simulink model "BEVplantModel"  (R2022b)
settings: Solver=daessc  StartTime=0  StopTime=50  RelTol=1e-3
PreLoadFcn:
  | % Load all parameters
  | BEVplantModelParam;
undefined symbols (not defined in the file): battery, cabin_T_init, coolant_pipe_D, coolant_valve_D_ratio_max, coolant_valve_D_ratio_min, coolant_valve_displacement, electricDrive, max_torque, vehicle, vehicleThermal
libraries: fl_lib x292, nesl_utility x67, SimscapeFluids_lib x15, ee_lib x11, sdl_lib x8, BatteryCurrentManagement x3, slpidlib x3, simulink x2, BatteryThermalManagement x1, autolibshared x1
(part 1 of 10)
Description:
  | Copyright 2022 - 2023 The MathWorks, Inc.
settings Model: PauseTimes=0.4  Creator=jjha  LastModifiedBy=jjha
settings SolverCC: ZeroCrossAlgorithm=Adaptive  DecoupledContinuousIntegration=on
settings DataIOCC: Decimation=10  ReturnWorkspaceOutputs=off  ReturnWorkspaceOutputsName=SimlogBEVdata
settings DebuggingCC: IgnoredZcDiagnostic=none
settings SimscapeCC: SimscapeLogType=all  SimscapeLogSimulationStatistics=on  SimscapeLogToSDI=on  SimscapeLogName=simlogBevPlantModel  SimscapeLogDecimation=10  SimscapeLogLimitData=off

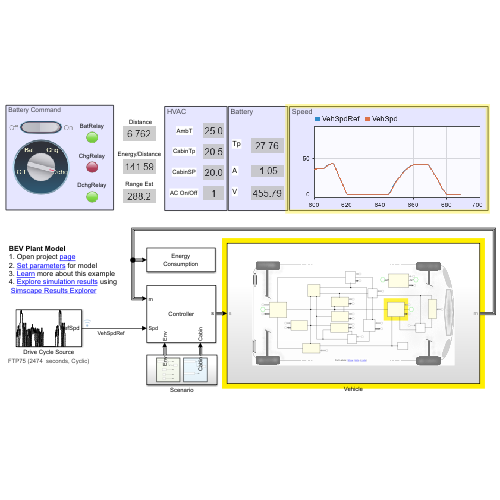
[thumbnail: Simulink's stored preview of the top-level diagram]
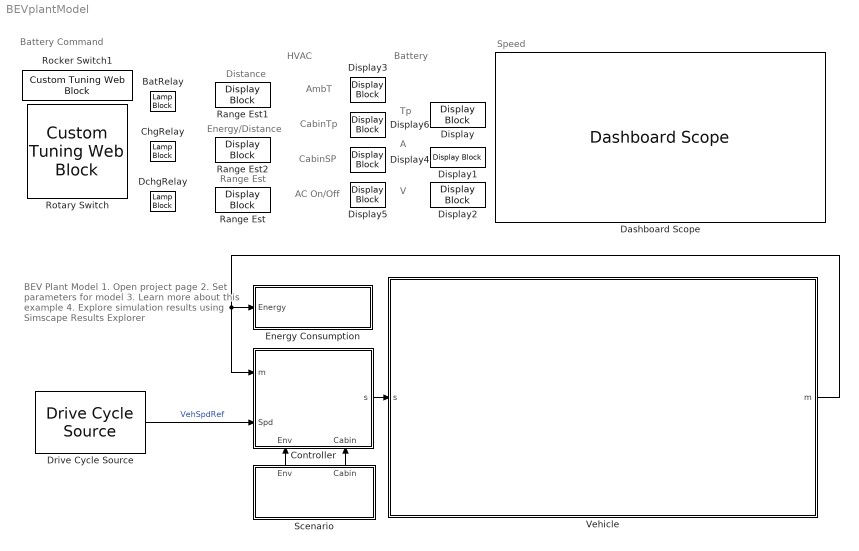
== system BEVplantModel ==
  note: BEV Plant Model
      | 1. Open project page
      | 2. Set parameters for model
      | 3. Learn more about this example
      | 4. Explore simulation results using
      | Simscape Results Explorer
  note: AC On/Off
  note: CabinSP
  note: AmbT
  note: Range Est
  note: HVAC
  note: Tp
  note: Battery
  note: Speed
  note: A
  note: V
  note: CabinTp
  note: Distance
  note: Energy/Distance
  note: Battery Command
  BatRelay : LampBlock  LabelPosition=Hide
  ChgRelay : LampBlock  LabelPosition=Hide
  Controller : Subsystem
      settings: PortSchema="{\"entries\":[{\"content\":{\"sides\":[{\"content\":{\"connectorIds\":[\"In1\",\"In2\"]},\"type\":\"ConnectorPlacement.EquallySpacedRectSide\",\"uuid\":\"c1a23be5-b2bd-489c-89d3-d8ff166adbae\"},{\"content\":{\"connectorIds\":[\"Out1\"],\"side\":\"RIGHT\"},\"type\":\"ConnectorPlacement.EquallySpacedRectSide\",\"uuid\":\"158e6e89-d1bb-4c90-8b36-55bfa29ba4ac\"},{\"content\":{\"connectorIds\":[],\"side\":\"TOP\"},\"type\":\"ConnectorPlacement.EquallySpacedRectSide\",\"uuid\":\"911e2005-fcf6-44eb-a0ec-ba245b30b3ee\"},{\"content\":{\"connectorIds\":[\"In3\",\"In4\"],\"side\":\"BOTTOM\"},\"type\":\"ConnectorPlacement.EquallySpacedRectSide\",\"uuid\":\"99a46f53-b2c3-4e95-9f3e-50b925639021\"}]},\"type\":\"ConnectorPlacement.EquallySpacedConnector\",\"uuid\":\"b6f9d50f-1ffb-42a1-8725-4930e4702b55\"}],\"packageUris\":[\"http://schema.mathworks.com/mf0/Connector/R2020b\"],\"version\":\"1.0\"}"
      mask Display: disp(get_param(gcb, 'Name'))
  Dashboard Scope : DashboardScope  Ymin=0  Ymax=150
  DchgRelay : LampBlock  LabelPosition=Hide
  Display : DisplayBlock  LabelPosition=Hide  Format=Custom  Transparency=1  FormatString=%.2f
  Display1 : DisplayBlock  LabelPosition=Hide  Format=Custom  Transparency=1  FormatString=%.2f
  Display2 : DisplayBlock  LabelPosition=Hide  Format=Custom  Transparency=1  FormatString=%.2f
  Display3 : DisplayBlock  LabelPosition=Hide  Format=Custom  Transparency=1  FormatString=%.1f
  Display4 : DisplayBlock  LabelPosition=Hide  Format=Custom  Transparency=1  FormatString=%.1f
  Display5 : DisplayBlock  LabelPosition=Hide  Format=Integer  Transparency=1  FormatString=%.2f
  Display6 : DisplayBlock  LabelPosition=Hide  Format=Custom  Transparency=1  FormatString=%.1f
  Drive Cycle Source : autolibshared/Drive Cycle Source  cycleVar=FTP75  wsVar=DriveCycleEPA  fileVar=cycleFTP75.mat  tfinal="2474  seconds, Cyclic"  cycleRepeat=on  outAccPort=off  outGearPort=off  gearList=No gear data  t_wot1=5  xdot_woto=0  xdot_wot1=30  t_wot2=20  xdot_wot2=0  t_wotend=30  srcUnit=m/s  outUnit=km/h  srcAccUnit=m/s/s  outAccUnit=m/s^2  dt=0  aMode=1  faultOption=off  velBnd=2  velBndUnit=mph  inUnit=m/s  timeBnd=1  failOption=off  stopSim=off  maxFaultCnt=10  maxFaultTime=2  maxTotFaultTime=15  traceOption=off  dtTrace=1  traceWindow=10  lastDCname=FTP75  lastOutUnit=mph  lastDT=0  lastTB=1  lastSB=2  forceCalcBound=off
  Energy Consumption : Subsystem
      mask Display: disp(get_param(gcb, 'Name'))
  Range Est : DisplayBlock  LabelPosition=Hide  Format=Custom  Transparency=1  FormatString=%.1f
  Range Est1 : DisplayBlock  LabelPosition=Hide  Format=Custom  Transparency=1  FormatString=%.3f
  Range Est2 : DisplayBlock  LabelPosition=Hide  Format=Custom  Transparency=1  FormatString=%.2f
  Rocker Switch1 : CustomTuningWebBlock  LabelPosition=Hide  ShowInitialText=on  Configuration="{\"components\":[{\"name\":\"CustomSwitchStateComponent\",\"settings\":{\"position\":[0,0,1,1],\"states\":[{\"HitRegion\":{\"position\":[0,0,0.5,1]},\"Image\":{\"position\":[0.13,0,1,0.75],\"size\":[1,0.75],\"src\":\"data:image\\/svg+xml;base64,PHN2ZyB4bWxucz0iaHR0cDovL3d3dy53My5vcmcvMjAwMC9zdmciIHhtbG5zOnhsaW5rPSJodHRwOi8vd3d3LnczLm9yZy8xOTk5L3hsaW5rIiB2aWV3Qm94PSIwIDAgNzUgMjQuOCI+PGRlZnM+PHN0eWxlPi5jbHMtMXtmaWxsOnVybCgjcmFkaWFsLWdyYWRpZW50KTt9LmNscy0ye2ZpbGw6dXJsKCNyYWRpYWwtZ3JhZGllbnQtMik7fS5jbHMtM3tzdHJva2U6I2IyMDAwMDtzdHJva2Utd2lkdGg6MC4yNXB4O2ZpbGw6dXJsKCNsaW5lYXItZ3JhZGllbnQpO30uY2xzLTR7ZmlsbDp1cmwoI2xpbmVhci1ncmFkaWVudC0yKTt9LmNs ...(+3576 chars)\",\"srcOrientation\":\"Right\"},\"Label\":{\"color\":[0.5019607843137255,0.5019607843137255,0.5019607843137255],\"icon\":{\"size\":[0,0],\"src\":[],\"srcOrientation\":\"Right\"},\"iconPlacement\":\"left\",\"opacity\":1,\"position\":[0.5,0.08],\"show\":true,\"text\":{\"content\":\"Off\",\"font\":\"Helvetica\",\"fontSize\":14}},\"Value\":0},{\"HitRegion\":{\"position\":[0,0.5,0.5,1]},\"Image\":{\"position\":[0.13,0,1,0.75],\"size\":[1,0.75],\"src\":\"data:image\\/svg+xml;base64,PHN2ZyB4bWxucz0iaHR0cDovL3d3dy53My5vcmcvMjAwMC9zdmciIHhtbG5zOnhsaW5rPSJodHRwOi8vd3d3LnczLm9yZy8xOTk5L3hsaW5rIiB2aWV3Qm94PSIwIDAgNzUgMjQuOCI+PGRlZnM+PHN0eWxlPi5jbHMtMXtmaWxsOnVybCgjcmFkaWFsLWdyYWRpZW50KTt9LmNscy0ye2ZpbGw6dXJsKCNyYWRpYWwtZ3JhZGllbnQtMik7fS5jbHMtM3tzdHJva2U6I2IyMDAwMDtzdHJva2Utd2lkdGg6MC4yNXB4O2ZpbGw6dXJsKCNsaW5lYXItZ3JhZGllbnQpO30uY2xzLTR7ZmlsbDp1cmwoI2xpbmVhci1ncmFkaWVudC0yKTt9LmNs ...(+3520 chars)\",\"srcOrientation\":\"Right\"},\"Label\":{\"color\":[0.5019607843137255,0.5019607843137255,0.5019607843137255],\"icon\":{\"size\":[0,0],\"src\":[],\"srcOrientation\":\"Right\"},\"iconPlacement\":\"left\",\"opacity\":1,\"position\":[0.5,0.92],\"show\":true,\"text\":{\"content\":\"On\",\"font\":\"Helvetica\",\"fontSize\":14}},\"Value\":1}]}},{\"name\":\"BackgroundImageComponent\",\"settings\":{\"image\":{\"size\":[155,70],\"src\":\"default\",\"srcOrientation\":\"Right\"},\"position\":[0,0,1,1],\"scaleMode\":\"0\"}},{\"name\":\"ForegroundImageComponent\",\"settings\":{\"image\":{\"size\":[0,0],\"src\":\"default\",\"srcOrientation\":[]},\"isForeground\":1,\"position\":[0,0,1,1],\"scaleMode\":\"0\"}}],\"settings\":{\"BindingType\":\"param\",\"backgroundColor\":[0,0,255,\"1\"],\"backgroundOffset\":0.14,\"fixedAspectRatio\":\"on\",\"foregroundColor\":[234,234,234],\"showBackgroundColor\":false,\"variant\":\"rocker\",\"version\":\"R2022b\"},\"type\":\"Switch\"}"
  Rotary Switch : CustomTuningWebBlock  LabelPosition=Hide  ShowInitialText=on  Configuration="{\"components\":[{\"name\":\"RotarySwitchComponent\",\"settings\":{\"arcAngle\":210,\"arcAngleOffset\":165,\"handle\":{\"size\":[150,150],\"src\":\"data:image\\/svg+xml;base64,PHN2ZyBpZD0iTGF5ZXJfMSIgZGF0YS1uYW1lPSJMYXllciAxIiB4bWxucz0iaHR0cDovL3d3dy53My5vcmcvMjAwMC9zdmciIHhtbG5zOnhsaW5rPSJodHRwOi8vd3d3LnczLm9yZy8xOTk5L3hsaW5rIiB2aWV3Qm94PSIwIDAgMTIxIDEyMSI+PGRlZnM+PHN0eWxlPi5jbHMtMXtmaWxsOnVybCgjbGluZWFyLWdyYWRpZW50KTt9LmNscy0yLC5jbHMtM3tmaWxsOiNkMWQxZDE7fS5jbHMtM3tzdHJva2U6I2I3YjdiNztzdHJva2UtbWl0ZXJsaW1pdDoxMDtzdHJva2Utd2lkdGg6MC4yNXB4O30uY2xzLTR7ZmlsbDojZjMwMDAwO30uY2xzLTV7ZmlsbDojZjIxNzY3O308L3N0eWxlPjxsaW5lYXJHcmFkaWVudCBpZD0ibGluZWFyLWdyYWRpZW50IiB4MT0iNjAuNSIgeTE9IjEyMC41IiB4Mj0iNjAuNSIgeTI9IjAuNSIgZ3JhZGllbnRVbml0cz0idXNlclNwYWNlT25Vc2UiPjxzdG9wIG9mZnNldD0iMCIgc3RvcC1jb2xvcj0iI2QxZDFkMSIvPjxzdG9wIG9mZnNldD0iMC4xIiBzdG9wLWNvbG9yPSIjY2VjZWNlIi8+PHN0b3Agb2Zmc2V0PSIwLjE5IiBzdG9wLWNvbG9yPSIjYzNjM2MzIi8+PHN0b3Agb2Zmc2V0PSIwLjI4IiBzdG9wLWNvbG9yPSIjYjFiMWIxIi8+PHN0b3Agb2Zmc2V0PSIwLjM2IiBzdG9wLWNvbG9yPSIjOTg5ODk4Ii8+PHN0b3Agb2Zmc2V0PSIwLjQ0IiBzdG9wLWNvbG9yPSIjNzg3ODc4Ii8+PHN0b3Agb2Zmc2V0PSIwLjQ2IiBzdG9wLWNvbG9yPSIjNmI2YjZiIi8+PHN0b3Agb2Zmc2V0PSIwLjU0IiBzdG9wLWNvbG9yPSIjNmI2YjZiIi8+PHN0b3Agb2Zmc2V0PSIwLjU2IiBzdG9wLWNvbG9yPSIjNzY3Njc2Ii8+PHN0b3Agb2Zmc2V0PSIwLjY0IiBzdG9wLWNvbG9yPSIjOTc5Nzk3Ii8+PHN0b3Agb2Zmc2V0PSIwLjcyIiBzdG9wLWNvbG9yPSIjYjBiMGIwIi8+PHN0b3Agb2Zmc2V0PSIwLjgxIiBzdG9wLWNvbG9yPSIjYzNjM2MzIi8+PHN0b3Agb2Zmc2V0PSIwLjkiIHN0b3AtY29sb3I9IiNjZGNkY2QiLz48c3RvcCBvZmZzZXQ9IjEiIHN0b3AtY29sb3I9IiNkMWQxZDEiLz48L2xpbmVhckdyYWRpZW50PjwvZGVmcz48Y2lyY2xlIGNsYXNzPSJjbHMtMSIgY3g9IjYwLjUiIGN5PSI2MC41IiByPSI2MCIvPjxwYXRoIGNsYXNzPSJjbHMtMiIgZD0iTTYwLjUsMUE1OS41LDU5LjUsMCwxLDEsMSw2MC41LDU5LjU3LDU5LjU3LDAsMCwxLDYwLjUsMW0wLTFBNjAuNSw2MC41LDAsMSwwLDEyMSw2MC41LDYwLjUsNjAuNSwwLDAsMCw2MC41LDBaIi8+PHJlY3QgY2xhc3M9ImNscy0zIiB4PSIwLjUiIHk9IjUxLjUiIHdpZHRoPSIxMjAiIGhlaWdodD0iMTgiIHJ4PSIzLjA0Ii8+PHJlY3QgY2xhc3M9ImNscy00IiB4PSI1Ljc1IiB5PSI1OC43NSIgd2lkdGg9IjE2IiBoZWlnaHQ9IjMiLz48cGF0aCBjbGFzcz0iY2xzLTUiIGQ9Ik0yMS4yNSw1OS4yNXYyaC0xNXYtMmgxNW0xLTFoLTE3djRoMTd2LTRaIi8+PC9zdmc+\"},\"handleOffset\":[0,0],\"handleOrientation\":180,\"handlePosition\":[0,0,1,1],\"handleSize\":{\"height\":0.5,\"width\":0.5},\"labelRadius\":0.36,\"position\":[0,0,1,1],\"states\":[{\"Label\":{\"color\":[0,0,0,1],\"icon\":{\"size\":[0,0],\"src\":[],\"srcOrientation\":\"Right\"},\"iconPlacement\":\"left\",\"opacity\":1,\"position\":[0.7345552884615385,0.6796274038461538],\"show\":true,\"text\":{\"content\":\"Off\",\"font\":\"Helvetica\",\"fontSize\":24}},\"Value\":0},{\"Label\":{\"color\":[0,0,0,1],\"icon\":{\"size\":[0,0],\"src\":[],\"srcOrientation\":\"Right\"},\"iconPlacement\":\"left\",\"opacity\":1,\"position\":[0.35757211538461536,0.7603966346153846],\"show\":true,\"text\":{\"content\":\"Bat\",\"font\":\"Helvetica\",\"fontSize\":24}},\"Value\":1},{\"Label\":{\"color\":[0,0,0,1],\"icon\":{\"size\":[0,0],\"src\":[],\"srcOrientation\":\"Right\"},\"iconPlacement\":\"left\",\"opacity\":1,\"position\":[0.09603365384615385,0.46033653846153844],\"show\":true,\"text\":{\"content\":\"Chg\",\"font\":\"Helvetica\",\"fontSize\":24}},\"Value\":2},{\"Label\":{\"color\":[0,0,0,1],\"icon\":{\"size\":[0,0],\"src\":[],\"srcOrientation\":\"Right\"},\"iconPlacement\":\"left\",\"opacity\":1,\"position\":[0.36532451923076925,0.1180889423076923],\"show\":true,\"text\":{\"content\":\"Dchg\",\"font\":\"Helvetica\",\"fontSize\":24}},\"Value\":3}],\"tickRadius\":0.32}},{\"name\":\"BackgroundImageComponent\",\"settings\":{\"image\":{\"size\":[155,150],\"src\":\"data:image\\/svg+xml;base64,PD94bWwgdmVyc2lvbj0iMS4wIiBlbmNvZGluZz0idXRmLTgiPz4NCjwhLS0gR2VuZXJhdG9yOiBBZG9iZSBJbGx1c3RyYXRvciAyNS4wLjAsIFNWRyBFeHBvcnQgUGx1Zy1JbiAuIFNWRyBWZXJzaW9uOiA2LjAwIEJ1aWxkIDApICAtLT4NCjxzdmcgdmVyc2lvbj0iMS4xIg0KCSBpZD0iTGF5ZXJfMl8xXyIgeG1sbnM6Y2M9Imh0dHA6Ly9jcmVhdGl2ZWNvbW1vbnMub3JnL25zIyIgeG1sbnM6ZGM9Imh0dHA6Ly9wdXJsLm9yZy9kYy9lbGVtZW50cy8xLjEvIiB4bWxuczppbmtzY2FwZT0iaHR0cDovL3d3dy5pbmtzY2FwZS5vcmcv ...(+4184 chars)\",\"srcOrientation\":\"Right\"},\"position\":[0,0,1,1],\"scaleMode\":\"0\"}},{\"name\":\"ForegroundImageComponent\",\"settings\":{\"image\":{\"size\":[0,0],\"src\":\"default\",\"srcOrientation\":[]},\"isForeground\":1,\"position\":[0,0,1,1],\"scaleMode\":\"0\"}}],\"settings\":{\"BindingType\":\"param\",\"backgroundColor\":[0,0,255,\"1\"],\"backgroundOffset\":1,\"enumDataType\":\"\",\"fixedAspectRatio\":\"on\",\"image\":{\"size\":[150,150],\"src\":\"data:image\\/svg+xml;base64,PD94bWwgdmVyc2lvbj0iMS4wIiBlbmNvZGluZz0iVVRGLTgiIHN0YW5kYWxvbmU9Im5vIj8+CjwhLS0gR2VuZXJhdG9yOiBBZG9iZSBJbGx1c3RyYXRvciAxOS4yLjEsIFNWRyBFeHBvcnQgUGx1Zy1JbiAuIFNWRyBWZXJzaW9uOiA2LjAwIEJ1aWxkIDApICAtLT4KCjxzdmcKICAgeG1sbnM6ZGM9Imh0dHA6Ly9wdXJsLm9yZy9kYy9lbGVtZW50cy8xLjEvIgogICB4bWxuczpjYz0iaHR0cDovL2NyZWF0aXZlY29tbW9ucy5vcmcvbnMjIgogICB4bWxuczpyZGY9Imh0dHA6Ly93d3cudzMub3JnLzE5OTkvMDIvMjItcmRmLXN5bnRh ...(+9660 chars)\"},\"showBackgroundColor\":false,\"useEnumDataType\":false,\"variant\":\"rotarySwitch\",\"version\":\"R2022b\"},\"type\":\"RotarySwitch\"}"
  Scenario : Subsystem  Tag=cold weather
      settings: PortSchema="{\"entries\":[{\"content\":{\"sides\":[{\"content\":{\"connectorIds\":[]},\"type\":\"ConnectorPlacement.EquallySpacedRectSide\",\"uuid\":\"eb8d1f37-8208-4a35-a227-ee3e7712aac0\"},{\"content\":{\"connectorIds\":[],\"side\":\"RIGHT\"},\"type\":\"ConnectorPlacement.EquallySpacedRectSide\",\"uuid\":\"04c1ce39-a668-46a3-bb9a-590d9fa6d188\"},{\"content\":{\"connectorIds\":[\"Out1\",\"Out2\"],\"side\":\"TOP\"},\"type\":\"ConnectorPlacement.EquallySpacedRectSide\",\"uuid\":\"9d96e5e2-2b9d-42e1-9359-7f2aa762ed32\"}]},\"type\":\"ConnectorPlacement.EquallySpacedConnector\",\"uuid\":\"d1c4a0ed-0ab9-4caa-880d-25dbcbc152ad\"}],\"packageUris\":[\"http://schema.mathworks.com/mf0/Connector/R2020b\"],\"version\":\"1.0\"}"
  Vehicle : Subsystem
  wires:
  Controller/1(s) -> Vehicle/1(s)
  Vehicle/1(m) -> Controller/1(m), Energy Consumption/1(Energy)
  Drive Cycle Source/1 -> Controller/2(Spd)  "VehSpdRef"
  Scenario/1(Env) -> Controller/3(Env)
  Scenario/2(Cabin) -> Controller/4(Cabin)

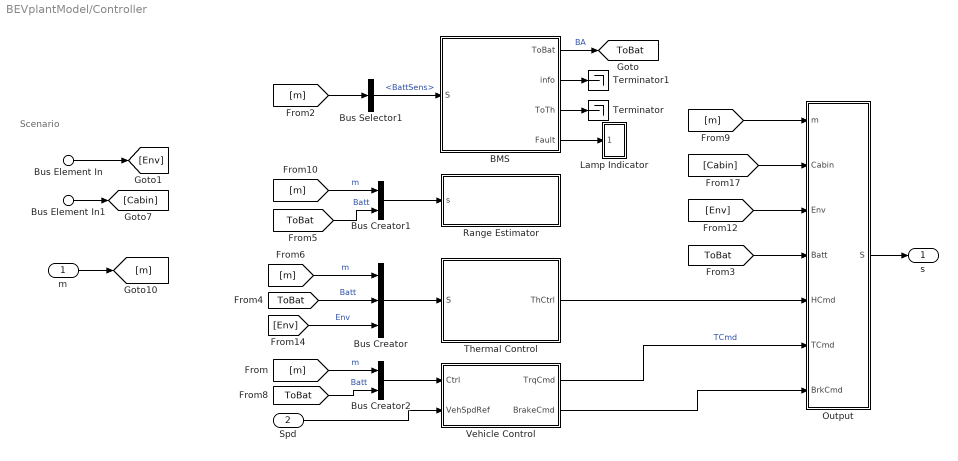
== system BEVplantModel/Controller ==
  note: Scenario
  m : Inport
  Spd : Inport  Port=2
  Bus Element In : Inport  Port=3  PortName=Env
  Bus Element In1 : Inport  Port=4  PortName=Cabin
  BMS : Subsystem
      settings: PortSchema="{\"entries\":[{\"content\":{\"sides\":[{\"content\":{\"connectorIds\":[]},\"type\":\"ConnectorPlacement.EquallySpacedRectSide\",\"uuid\":\"92c05094-f9b0-45a3-ac1b-1858c0c996e8\"},{\"content\":{\"connectorIds\":[],\"side\":\"RIGHT\"},\"type\":\"ConnectorPlacement.EquallySpacedRectSide\",\"uuid\":\"cdc13757-7d0c-4e35-a976-de64c06d8cde\"},{\"content\":{\"connectorIds\":[\"In1\"],\"side\":\"TOP\"},\"type\":\"ConnectorPlacement.EquallySpacedRectSide\",\"uuid\":\"c53a1ad0-a5f6-468e-b5dd-f0a27cee9942\"},{\"content\":{\"connectorIds\":[\"Out1\",\"Out2\",\"Out3\",\"Out4\"],\"side\":\"BOTTOM\"},\"type\":\"ConnectorPlacement.EquallySpacedRectSide\",\"uuid\":\"8abfd502-0389-4393-bb18-f131709acb23\"}]},\"type\":\"ConnectorPlacement.EquallySpacedConnector\",\"uuid\":\"102d552e-f167-4796-a536-13938ac07fac\"}],\"packageUris\":[\"http://schema.mathworks.com/mf0/Connector/R2020b\"],\"version\":\"1.0\"}"
  Bus Creator : BusCreator  Inputs=3
  Bus Creator1 : BusCreator  Inputs=2
  Bus Creator2 : BusCreator  Inputs=2
  Bus Selector1 : BusSelector  OutputSignals=BA.BattSens
  Lamp Indicator : Subsystem
      settings: PortSchema="{\"entries\":[{\"content\":{\"sides\":[{\"content\":{\"connectorIds\":[]},\"type\":\"ConnectorPlacement.EquallySpacedRectSide\",\"uuid\":\"c55e4a0c-c727-4224-8aa6-2961c151763f\"},{\"content\":{\"connectorIds\":[],\"side\":\"RIGHT\"},\"type\":\"ConnectorPlacement.EquallySpacedRectSide\",\"uuid\":\"62aa4b95-0b95-454c-8041-b3e5f6582f45\"},{\"content\":{\"connectorIds\":[\"In1\"],\"side\":\"TOP\"},\"type\":\"ConnectorPlacement.EquallySpacedRectSide\",\"uuid\":\"0d235e8c-306c-4ade-b7e4-bd2fcf6610c8\"}]},\"type\":\"ConnectorPlacement.EquallySpacedConnector\",\"uuid\":\"6725a8d5-e875-410a-8026-694fde1b795b\"}],\"packageUris\":[\"http://schema.mathworks.com/mf0/Connector/R2020b\"],\"version\":\"1.0\"}"
  Output : Subsystem
  Range Estimator : Subsystem
  Terminator : Terminator
  Terminator1 : Terminator
  Thermal Control : Subsystem
  Vehicle Control : Subsystem
  s : Outport
  tag scope: ToBat=global
  wires:
  [m] -> Bus Creator/1  "m"
  Bus Creator/1 -> Thermal Control/1(S)
  [ToBat] -> Bus Creator1/2  "Batt"
  Thermal Control/1(ThCtrl) -> Output/5(HCmd)
  [Env] -> Bus Creator/3  "Env"
  Vehicle Control/1(TrqCmd) -> Output/6(TCmd)  "TCmd"
  Bus Selector1/1 -> BMS/1(S)  "<BattSens>"
  BMS/2(info) -> Terminator1/1
  BMS/4(Fault) -> Lamp Indicator/1(" ")
  BMS/3(ToTh) -> Terminator/1
  BMS/1(ToBat) -> [ToBat]  "BA"
  Spd/1 -> Vehicle Control/2(VehSpdRef)
  m/1 -> [m]
  Vehicle Control/2(BrakeCmd) -> Output/7(BrkCmd)
  Output/1(S) -> s/1
  [ToBat] -> Output/4(Batt)
  [Env] -> Output/3(Env)
  [Cabin] -> Output/2(Cabin)
  Bus Element In/1 -> [Env]
  Bus Element In1/1 -> [Cabin]
  Bus Creator1/1 -> Range Estimator/1(s)
  [ToBat] -> Bus Creator/2  "Batt"
  [ToBat] -> Bus Creator2/2  "Batt"
  Bus Creator2/1 -> Vehicle Control/1(Ctrl)
  [m] -> Bus Creator2/1  "m"
  [m] -> Bus Selector1/1
  [m] -> Output/1(m)
  [m] -> Bus Creator1/1  "m"

== system BEVplantModel/Energy Consumption ==
  Bus Element In : Inport  PortName=Energy
  Add : Sum  Inputs=++++
  Aux Energy : Subsystem
  Bus Selector : BusSelector  OutputSignals=M2.EM2energy,M1.EM1energy,VA.HVACenergy
  Bus Selector1 : BusSelector  OutputSignals=MP.MotorPumpCurr,BP.BattPumpCurr,MP.LowVolt,HE.HeaterCurrent,CH.ChillerCurrent,BA.BattSens.Cellvolt
  Display{,1..4} (5 alike) : Display
  Sum : Sum
  Sum of Elements : Sum  Inputs=+
  Sum1 : Sum
  wires:
  [EM2energy] -> Add/2
  [EM1energy] -> Add/3
  [HVACenergy] -> Add/4
  Add/1 -> Display/1  "EnergyCons"
  Aux Energy/1(E) -> Display1/1, Add/1  "AuxEnergy"
  [EM2energy] -> Display2/1  "EM2energy"
  [EM1energy] -> Display3/1  "EM1energy"
  [HVACenergy] -> Display4/1  "HVACenergy"
  Bus Selector/1 -> [EM2energy]  "<EM2energy>"
  Bus Selector/2 -> [EM1energy]  "<EM1energy>"
  Bus Selector/3 -> [HVACenergy]  "<HVACenergy>"
  Bus Element In/1 -> Bus Selector/1, Bus Selector1/1
  Bus Selector1/5 -> Sum/2  "<ChillerCurrent>"
  Bus Selector1/3 -> Aux Energy/2(LowVolt)  "<LowVolt>"
  Sum1/1 -> Aux Energy/1(AuxLoCur)
  Sum/1 -> Aux Energy/3(AuxHiCur)
  Bus Selector1/4 -> Sum/1  "<HeaterCurrent>"
  Bus Selector1/1 -> Sum1/1  "<MotorPumpCurr>"
  Bus Selector1/2 -> Sum1/2  "<BattPumpCurr>"
  Bus Selector1/6 -> Sum of Elements/1  "<Cellvolt>"
  Sum of Elements/1 -> Aux Energy/4(BattVolt)

== system BEVplantModel/Scenario ==
  note: Cabin HVAC
  note: Environment
  AC On/Off : Constant  Value=vehicleThermal.AConoff
  CO2 Fraction : Constant  Value=4e-4
  Display : Display
  Display1 : Display
  K to degC : Subsystem
  K to degC1 : Subsystem
  Pressure [MPa] : Constant  Value=0.101325
  Relative Humidity : Constant  Value=0.5
  Temperature Setpoint [K] : Constant  Value=vehicleThermal.CabinSpTp
  Temperature [K] : Constant  Value=vehicleThermal.ambient
  Bus Element Out : Outport  PortName=Env  Element=Tenv
  Bus Element Out1 : Outport  PortName=Env  Element=Penv
  Bus Element Out2 : Outport  PortName=Env  Element=RHenv
  Bus Element Out3 : Outport  PortName=Env  Element=CO2env
  Bus Element Out4 : Outport  Port=2  PortName=Cabin  Element=TpSetPoint
  Bus Element Out5 : Outport  Port=2  PortName=Cabin  Element=acOnOff
  wires:
  Relative Humidity/1 -> Bus Element Out2/1
  AC On/Off/1 -> Bus Element Out5/1
  Temperature Setpoint [K]/1 -> K to degC1/1(" "), Bus Element Out4/1
  CO2 Fraction/1 -> Bus Element Out3/1
  Temperature [K]/1 -> Bus Element Out/1, K to degC/1(" ")
  Pressure [MPa]/1 -> Bus Element Out1/1
  K to degC/1("  ") -> Display/1
  K to degC1/1("  ") -> Display1/1
